simulink model "LADRC_Bloque_py_b"  (R2021a)
settings: Solver=ode8  StartTime=0.0  StopTime=10.0  FixedStep=0.01  RelTol=1e-3
settings Model: Creator=djah0  LastModifiedBy=djah0
settings DataIOCC: ReturnWorkspaceOutputs=off

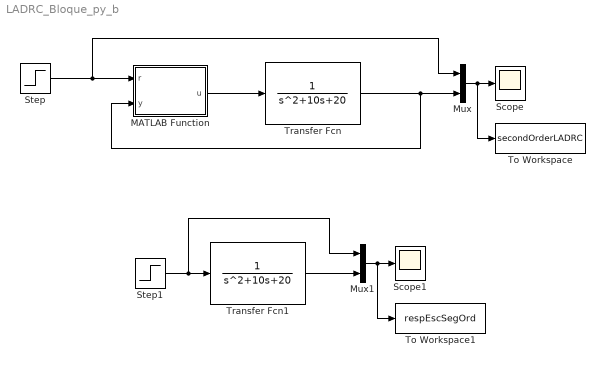
== system LADRC_Bloque_py_b ==
  MATLAB Function : MATLAB Function  TreatAsAtomicUnit=on
  Mux : Mux  Inputs=2
  Mux1 : Mux  Inputs=2
  Scope : Scope
  Scope1 : Scope
  Step : Step  SampleTime=0
  Step1 : Step  SampleTime=0
  To Workspace : ToWorkspace  VariableName=secondOrderLADRC  SaveFormat=Timeseries  SampleTime=-1
  To Workspace1 : ToWorkspace  VariableName=respEscSegOrd  SaveFormat=Timeseries  SampleTime=-1
  Transfer Fcn : TransferFcn  Denominator=[1 10 20]
  Transfer Fcn1 : TransferFcn  Denominator=[1 10 20]
  wires:
  MATLAB Function/1(u) -> Transfer Fcn/1
  Transfer Fcn/1 -> Mux/2, MATLAB Function/2(y)
  Step/1 -> Mux/1, MATLAB Function/1(r)
  Mux/1 -> To Workspace/1, Scope/1
  Transfer Fcn1/1 -> Mux1/2
  Step1/1 -> Mux1/1, Transfer Fcn1/1
  Mux1/1 -> To Workspace1/1, Scope1/1

== matlab function LADRC_Bloque_py_b/MATLAB Function ==
  data: r input; u output; y input
function u = pyLADRC_b(r, y)
%#codegen

u = 0; % Preasignado

coder.extrinsic('pythonLADRC');
%poner h = 0.001 y step de simul en 0.0005 o en 0.001 y 0.001 ode3
param.nx = 2;
param.b = 1;
param.wc = 8;
param.wo = 48;
param.zo = 0;

u = pythonLADRC(r, y, param);
